simulink model "L2_4_subsystem"  (R2025b)
settings: Solver=VariableStepAuto  StartTime=0.0  StopTime=5  RelTol=1e-3
settings Model: Creator=kimsteph  LastModifiedBy=kimsteph

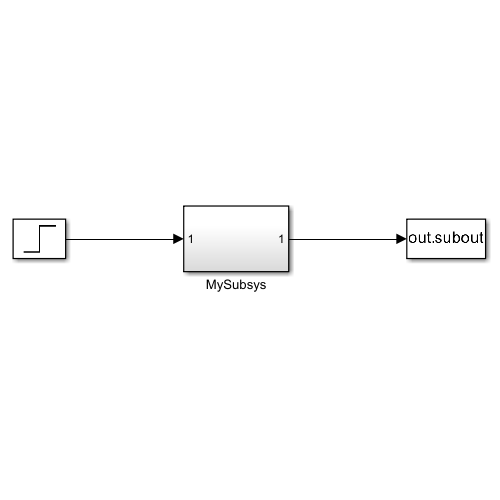
[thumbnail: Simulink's stored preview of the top-level diagram]
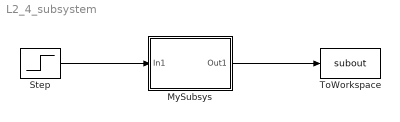
== system L2_4_subsystem ==
  MySubsys : Subsystem
  Step : Step  After=5  SampleTime=0
  ToWorkspace : ToWorkspace  VariableName=subout  SaveFormat=Timeseries  SampleTime=-1
  wires:
  Step/1 -> MySubsys/1(In1)
  MySubsys/1(Out1) -> ToWorkspace/1

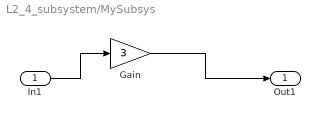
== system L2_4_subsystem/MySubsys ==
  In1 : Inport
  Gain : Gain  Gain=3
  Out1 : Outport
  wires:
  In1/1 -> Gain/1
  Gain/1 -> Out1/1
